simulink model "rapros"  (R2013a)
settings: Solver=FixedStepDiscrete  StartTime=0.0  StopTime=10  RelTol=1e-3
libraries: instrumentlib x2
settings Model: Creator=root  LastModifiedBy=root
settings SolverCC: AutoInsertRateTranBlk=on
settings DataIOCC: SignalLoggingSaveFormat=ModelDataLogs  SaveOutput=off  SaveTime=off
settings OptimizationCC: InlineParams=on  InlineInvariantSignals=on  StateBitsets=on  DataBitsets=on  UseTempVars=on  ZeroExternalMemoryAtStartup=off  ZeroInternalMemoryAtStartup=off  NoFixptDivByZeroProtection=on  OptimizeModelRefInitCode=on  LifeSpan=1
settings DebuggingCC: MultiTaskDSMMsg=warning  MultiTaskCondExecSysMsg=none  StrictBusMsg=None
settings HardwareCC: ProdIntDivRoundTo=Floor  ProdEndianess=LittleEndian  ProdHWDeviceType=Generic->Custom
settings RTWCC: SystemTargetFile=ert.tlc  TLCOptions=-p0  GenCodeOnly=on  TemplateMakefile=ert_default_tmf  Description=Embedded Coder  GenerateReport=on  RTWVerbose=off  ProcessScript=ert_make_rtw_hook  IncludeHyperlinkInReport=on  LaunchReport=on  IncludeERTFirstTime=on
settings CodeAppCC: ForceParamTrailComments=on  IgnoreCustomStorageClasses=off  SimulinkDataObjDesc=on  CustomSymbolStrGlobalVar=rt$N$M  CustomSymbolStrType=$N$M  CustomSymbolStrFcn=$N$M$F  CustomSymbolStrMacro=$N$M  InsertBlockDesc=on
settings ERTTargetCC: CodeReplacementLibrary=None  IncludeMdlTerminateFcn=off  SuppressErrorStatus=on  SupportAbsoluteTime=off  SupportNonFinite=off  SupportComplex=off  PurelyIntegerCode=on  RootIOFormat=Structure reference  ERTCustomFileTemplate=example_file_process.tlc

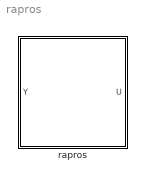
== system rapros ==
  rapros : Subsystem  mask{output_size=3, input_size=3, Ts=0.1, IP='127.0.0.1', IPs='127.0.0.1'}
      mask prompts: output_size "Input dimension"; input_size "Output dimesion"; Ts "Sample Time"; IP "Host address receive"; IPs "Host address send"
      mask init:
      | sys = get_param(0,'CurrentSystem');
      | input_size=[input_size 1];
      | datasize= mat2str(input_size);
      | ts= mat2str(Ts);
      | ip=IP;
      | Ip= mat2str(ip);
      | ips=IPs;
      | Ips= mat2str(ips);
      | set_param([sys '/rapros/Receive'],'DataSize',datasize);
      | set_param([sys '/rapros/Receive'],'Host',ip);
      | set_param([sys '/rapros/Receive'],'SampleTime',ts);
      | set_param([sys '/rapros/Send'],'Host',ips);

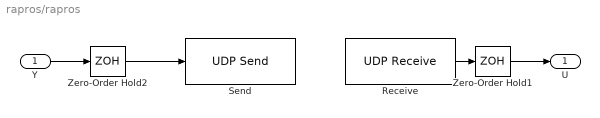
== system rapros/rapros ==
  Y : Inport  PortDimensions=output_size
  Receive : instrumentlib/UDP Receive  Priority=2  Host=127.0.0.1  Port=25000  LocalPort=667  DataSize=[3 1]  EnableBlockingMode=on  Timeout=1  SampleTime=0.1  DataType=double  ByteOrder=LittleEndian
  Send : instrumentlib/UDP Send  Priority=1  Host=127.0.0.1  Port=25001  LocalPort=666  EnableBlockingMode=on  ByteOrder=LittleEndian
  Zero-Order Hold1 : ZeroOrderHold  SampleTime=Ts
  Zero-Order Hold2 : ZeroOrderHold  SampleTime=Ts
  U : Outport
  wires:
  Y/1 -> Zero-Order Hold2/1
  Zero-Order Hold2/1 -> Send/1
  Zero-Order Hold1/1 -> U/1
  Receive/1 -> Zero-Order Hold1/1
